simulink model "lab4"  (Simulink 8.1)
settings: Solver=ode45  StartTime=0.0  StopTime=3  RelTol=1e-5
settings Model: Creator=srahili  LastModifiedBy=shwang
settings DebuggingCC: FcnCallInpInsideContextMsg=EnableAllAsWarning
settings GRTTargetCC: CombineOutputUpdateFcns=on  GRTInterface=off

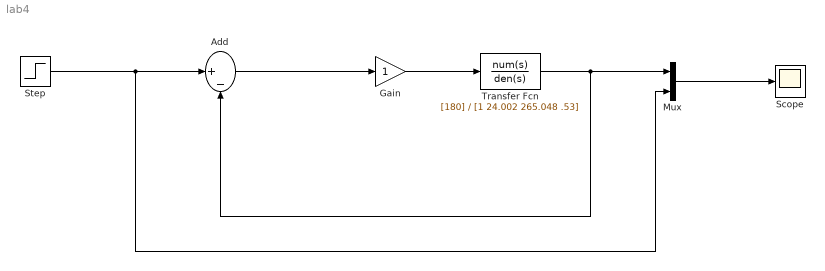
== system lab4 ==
  Add : Sum  Inputs=|+-
  Gain : Gain
  Mux : Mux  Inputs=2
  Scope : Scope
  Step : Step  Time=0  SampleTime=0
  Transfer Fcn : TransferFcn  Numerator=[180]  Denominator=[1 24.002 265.048 .53]
  wires:
  Step/1 -> Add/1, Mux/2
  Add/1 -> Gain/1
  Gain/1 -> Transfer Fcn/1
  Transfer Fcn/1 -> Mux/1, Add/2
  Mux/1 -> Scope/1
